simulink model "two_link_error"  (R2021a)
settings: Solver=VariableStepAuto  StartTime=0.0  StopTime=10.0  RelTol=1e-3
undefined symbols (not defined in the file or in its folder): F, f, K_D, K_P
settings Model: Creator=frida  LastModifiedBy=frida

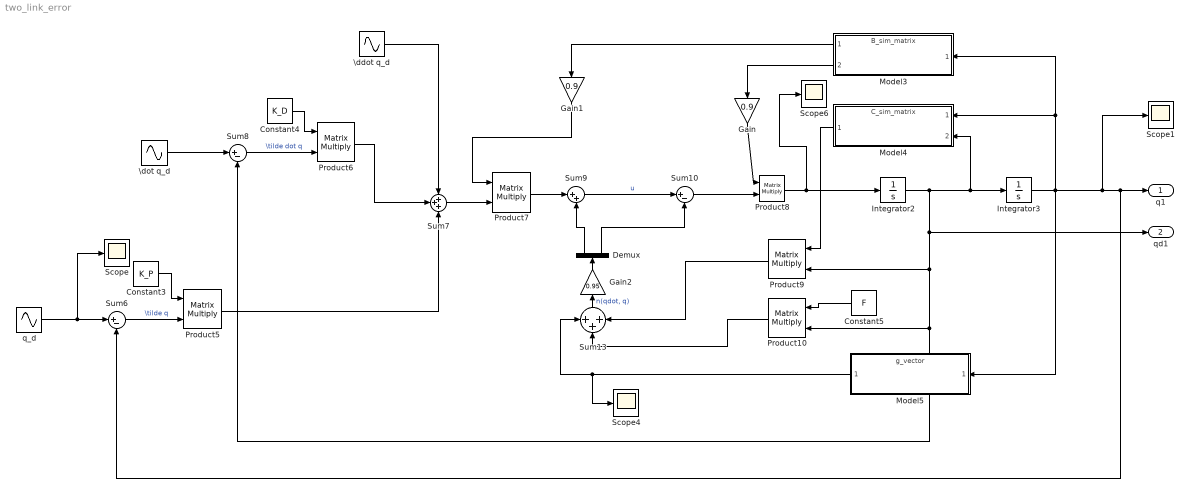
== system two_link_error ==
  Constant3 : Constant  Value=K_P
  Constant4 : Constant  Value=K_D
  Constant5 : Constant  Value=F
  Demux : Demux  Outputs=2
  Gain : Gain  Gain=0.9
  Gain1 : Gain  Gain=0.9
  Gain2 : Gain  Gain=0.95
  Integrator2 : Integrator
  Integrator3 : Integrator
  Model3 : ModelReference  ModelNameDialog=B_sim_matrix.slx  SimulationMode=Normal  ModelReferenceVersion=1.6
  Model4 : ModelReference  ModelNameDialog=C_sim_matrix.slx  SimulationMode=Normal  ModelReferenceVersion=1.2
  Model5 : ModelReference  ModelNameDialog=g_vector.slx  SimulationMode=Normal  ModelReferenceVersion=1.8
  Product{5..10} (6 alike) : Product  Multiplication=Matrix(*)
  Scope{,1,4,6} (4 alike) : Scope
  Sum10 : Sum  Inputs=|+-
  Sum13 : Sum  Inputs=+++
  Sum6 : Sum  Inputs=|+-
  Sum7 : Sum  Inputs=+++
  Sum8 : Sum  Inputs=|+-
  Sum9 : Sum  Inputs=|++
  \ddot q_d : Sin  Amplitude=-4*(pi^2)*(f^2)  Frequency=[2*pi*f, 2*pi*f]  SampleTime=0
  \dot q_d : Sin  Amplitude=2*pi*f  Frequency=[2*pi*f, 2*pi*f]  Phase=pi/2  SampleTime=0
  q_d : Sin  Frequency=[2*pi*f, 2*pi*f]  SampleTime=0
  q1 : Outport  PortDimensions=2
  qd1 : Outport  Port=2  PortDimensions=2
  wires:
  Sum10/1 -> Product8/2
  Sum9/1 -> Sum10/1  "u"
  Constant5/1 -> Product10/1
  Product8/1 -> Scope6/1, Integrator2/1
  Product10/1 -> Sum13/2
  Product9/1 -> Sum13/3
  q_d/1 -> Scope/1, Sum6/1
  Model3/1 -> Gain1/1
  Integrator2/1 -> Sum8/2, Product10/2, Product9/2, qd1/1, Model4/2, Integrator3/1
  Constant4/1 -> Product6/1
  Sum8/1 -> Product6/2  "\\tilde dot q"
  Model4/1 -> Product9/1
  Product7/1 -> Sum9/1
  Product5/1 -> Sum7/3
  Sum7/1 -> Product7/2
  Integrator3/1 -> Sum6/2, q1/1, Scope1/1, Model5/1, Model3/1, Model4/1
  \dot q_d/1 -> Sum8/1
  Product6/1 -> Sum7/2
  Model5/1 -> Scope4/1, Sum13/1
  \ddot q_d/1 -> Sum7/1
  Sum6/1 -> Product5/2  "\\tilde q"
  Constant3/1 -> Product5/1
  Model3/2 -> Gain/1
  Gain/1 -> Product8/1
  Gain1/1 -> Product7/1
  Demux/1 -> Sum9/2
  Sum13/1 -> Gain2/1  "n(qdot, q)"
  Gain2/1 -> Demux/1
  Demux/2 -> Sum10/2
